simulink model "sampleModel270"  (R2021b)
settings: Solver=VariableStepAuto  StartTime=0.0  StopTime=10.0  RelTol=1e-3
undefined symbols (not defined in the file or in its folder): DiscIntNeverNeededParam, Newton, Raphson
libraries: simulink x19, slpidlib x1
settings Model: Creator=user  LastModifiedBy=user

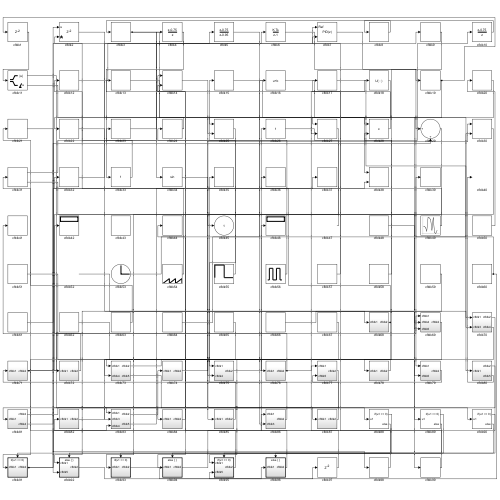
[thumbnail: Simulink's stored preview of the top-level diagram]
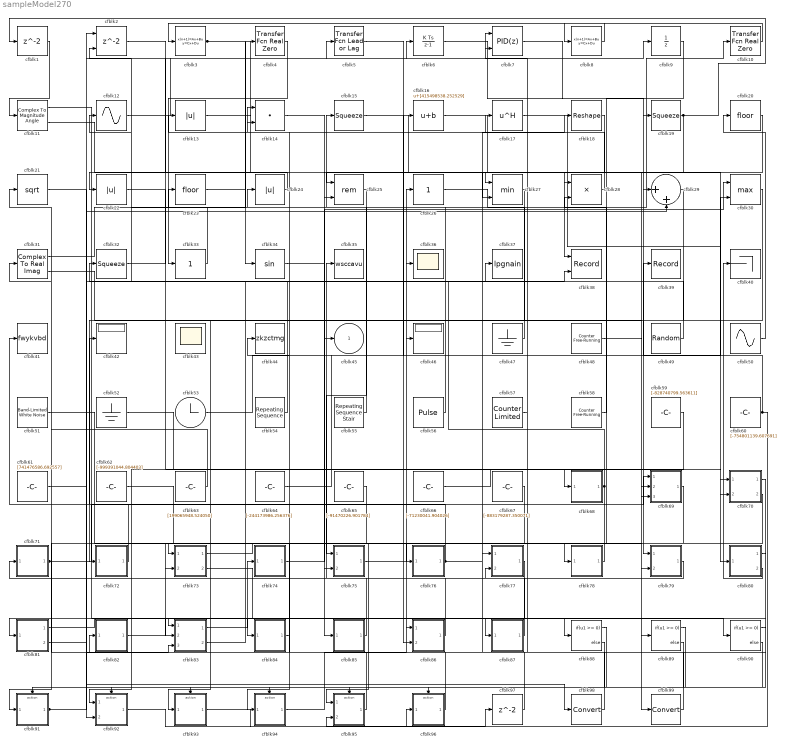
== system sampleModel270 ==
  cfblk1 : Delay  SampleTime=1
  cfblk10 : simulink/Discrete/Transfer Fcn Real Zero  ZeroZ=0.75  ICPrevInput=0.0  DoSatur=off
      settings: SourceProductBaseCode=SL
  cfblk11 : ComplexToMagnitudeAngle
  cfblk12 : Sin  TimeSource=Use external signal  SampleTime=0
  cfblk13 : Abs
  cfblk14 : DotProduct  InputSameDT=on  OutDataTypeStr=Inherit: Inherit via internal rule
  cfblk15 : Squeeze
  cfblk16 : Bias  Bias=[415498538.252529]
  cfblk17 : Math  Operator=hermitian  SaturateOnIntegerOverflow=on
  cfblk18 : Reshape
  cfblk19 : Squeeze
  cfblk2 : Delay  ShowEnablePort=on  SampleTime=1
      settings: InputPortMap=u0,e6
  cfblk20 : Rounding
  cfblk21 : Sqrt  SaturateOnIntegerOverflow=on
  cfblk22 : Abs
  cfblk23 : Rounding
  cfblk24 : Abs
  cfblk25 : Math  Operator=rem  SaturateOnIntegerOverflow=on
  cfblk26 : simulink/Math Operations/Slider Gain  gain=1  low=0  high=2
  cfblk27 : MinMax  Inputs=2
  cfblk28 : Product
  cfblk29 : Sum  Inputs=|++
  cfblk3 : DiscreteStateSpace
  cfblk30 : MinMax  Function=max  Inputs=2
  cfblk31 : ComplexToRealImag
  cfblk32 : Squeeze
  cfblk33 : simulink/Math Operations/Slider Gain  gain=1  low=0  high=2
  cfblk34 : Trigonometry
  cfblk35 : ToWorkspace  VariableName=wsccavu  SaveFormat=Timeseries  SampleTime=-1
  cfblk36 : Scope
  cfblk37 : ToWorkspace  VariableName=lpgnain  SaveFormat=Timeseries  SampleTime=-1
  cfblk38 : Record  FileSettingsInternal="{\"entries\":[{\"content\":{\"excelSettings\":{\"content\":{},\"type\":\"Streamout.ExcelSettings\"}},\"type\":\"Streamout.FileSettingStorage\",\"uuid\":\"55c07847-b416-4147-ba9b-c4fbf5457b55\"}],\"packageUris\":[\"http://schema.mathworks.com/mf0/streamout_blocks/R2020a\"],\"version\":\"1.0\"}"  Layout=[1 1]  SignalsInternal="{\"entries\":[{\"content\":{\"signals\":[{\"content\":{\"blockPath\":[\"sampleModel270/cfblk38\"],\"channel\":[],\"dimensions\":[1],\"domain\":\"sampleModel270/cfblk38\",\"lineColor\":\"#a2142f\",\"plots\":[1],\"port\":1,\"sid\":[\"\"],\"signalID\":11209,\"signalName\":\"cfblk16\"},\"type\":\"RecordBlkView.Signal\",\"uuid\":\"6d9d134b-09a8-4e77-b9a8-4c5e57516884\"},{\"content\":{\"blockPath\":[\"sampleModel270/cfblk38\"],\"channel\":[],\"dimensions\":[1],\"domain\":\"sampleModel270/cfblk38\",\"lineColor\":\"#139fff\",\"plots\":[1],\"port\":2,\"sid\":[\"\"],\"signalID\":11213,\"signalName\":\"cfblk91\"},\"type\":\"RecordBlkView.Signal\",\"uuid\":\"035bce28-8201-4e43-961c-4afa830852dc\"}]},\"type\":\"RecordBlkView.InputSignals\",\"uuid\":\"f20a0d1a-bcdb-4eb4-a0c7-2d20c3785a29\"}],\"packageUris\":[\"http://schema.mathworks.com/mf0/streamout_blocks/R2020a\"],\"version\":\"1.0\"}"  VisualizationBindings="{\"xyplotplugin\":{\"info\":[{\"series\":[{\"bindingParametersList\":[{\"parameter\":\"X-Axis\",\"signalID\":11209,\"signalName\":\"cfblk16\"},{\"parameter\":\"Y-Axis\",\"signalID\":11213,\"signalName\":\"cfblk91\"}],\"seriesID\":19260}],\"subplotID\":1}]}}"  CompatibilityTag=XY
  cfblk39 : Record  FileSettingsInternal="{\"entries\":[{\"content\":{\"excelSettings\":{\"content\":{},\"type\":\"Streamout.ExcelSettings\"}},\"type\":\"Streamout.FileSettingStorage\",\"uuid\":\"3d67d137-5401-4fa9-bcac-a18ba41f64ea\"}],\"packageUris\":[\"http://schema.mathworks.com/mf0/streamout_blocks/R2020a\"],\"version\":\"1.0\"}"  SignalsInternal="{\"entries\":[{\"content\":{\"signals\":[{\"content\":{\"blockPath\":[\"sampleModel270/cfblk39\"],\"channel\":[],\"dimensions\":[1],\"domain\":\"sampleModel270/cfblk39\",\"lineColor\":\"#fe330a\",\"plots\":[1],\"port\":1,\"sid\":[\"\"],\"signalID\":11217,\"signalName\":\"cfblk60\"},\"type\":\"RecordBlkView.Signal\",\"uuid\":\"4590cb18-5316-4242-95f9-f30dc2470911\"}]},\"type\":\"RecordBlkView.InputSignals\",\"uuid\":\"af798ec9-883d-434f-9e97-72437914e7d3\"}],\"packageUris\":[\"http://schema.mathworks.com/mf0/streamout_blocks/R2020a\"],\"version\":\"1.0\"}"  VisualizationBindings="{\"sparklinesplugin\":{\"info\":[{\"bindingParametersList\":[],\"subplotID\":1}]}}"
  cfblk4 : simulink/Discrete/Transfer Fcn Real Zero  ZeroZ=0.75  ICPrevInput=0.0  DoSatur=off
      settings: SourceProductBaseCode=SL
  cfblk40 : Terminator
  cfblk41 : ToWorkspace  VariableName=fwykvbd  SaveFormat=Timeseries  SampleTime=-1
  cfblk42 : Display
  cfblk43 : Scope
      settings: Floating=on
  cfblk44 : ToWorkspace  VariableName=zkzctmg  SaveFormat=Timeseries  SampleTime=-1
  cfblk46 : Display
  cfblk47 : Ground
  cfblk48 : simulink/Sources/Counter Free-Running  NumBits=[30.000000]  tsamp=-1
  cfblk49 : RandomNumber  Mean=[-13361.001595]  Variance=[83852.352686]  Seed=[353484768.000000]  SampleTime=0.1
  cfblk5 : simulink/Discrete/Transfer Fcn Lead or Lag  PoleZ=0.95  ZeroZ=0.75  ICPrevOutput=0.0  ICPrevInput=0.0  DoSatur=off
      settings: SourceProductBaseCode=SL
  cfblk50 : Sin  Amplitude=[595358799.977348]  Bias=[424544015.992801]  SampleTime=0
  cfblk51 : simulink/Sources/Band-Limited White Noise  Cov=[9502367799.789673]  Ts=0.1  seed=[5436201859.000000]
  cfblk52 : Ground
  cfblk53 : Clock
  cfblk54 : simulink/Sources/Repeating Sequence  rep_seq_t=[0 2]  rep_seq_y=[-647210942.038326, -486981734.967450]
  cfblk55 : simulink/Sources/Repeating Sequence Stair  OutValues=[958210710.074239, 342558910.444155]  tsamp=-1  OutMin=[]  OutMax=[]  OutDataTypeStr=double  OutputDataTypeScalingMode=double  OutDataType=fixdt(0,8)  ConRadixGroup=Best Precision: Vector-wise  OutScaling=2^-12
  cfblk56 : DiscretePulseGenerator  PulseType=Time based  Amplitude=[87379413.478695]  Period=[35675365.567741]  PulseWidth=5  PhaseDelay=[7.000000]
  cfblk57 : simulink/Sources/Counter Limited  uplimit=[460.000000]  tsamp=-1
  cfblk58 : simulink/Sources/Counter Free-Running  NumBits=[9.000000]  tsamp=-1
  cfblk59 : Constant  Value=[-828740799.563611]  SampleTime=1
  cfblk6 : DiscreteIntegrator  ICPrevOutput=DiscIntNeverNeededParam  ICPrevScaledInput=DiscIntNeverNeededParam
  cfblk60 : Constant  Value=[-754801139.607691]  SampleTime=1
  cfblk61 : Constant  Value=[741476586.692557]  SampleTime=1
  cfblk62 : Constant  Value=[-999391044.804403]  SampleTime=1
  cfblk63 : Constant  Value=[199065948.524050]  SampleTime=1
  cfblk64 : Constant  Value=[-244173986.256376]  SampleTime=1
  cfblk65 : Constant  Value=[-91470226.901784]  SampleTime=1
  cfblk66 : Constant  Value=[-71230041.904026]  SampleTime=1
  cfblk67 : Constant  Value=[-883179287.350071]  SampleTime=1
  cfblk68 : Subsystem
  cfblk69 : Subsystem
  cfblk7 : slpidlib/PID Controller (2DOF)  Controller=PID  Form=Parallel  TimeDomain=Discrete-time  UseExternalTs=off  SampleTime=1  IntegratorMethod=Forward Euler  FilterMethod=Forward Euler  ControllerParametersSource=internal  P=1  I=1  D=0  UseFilter=on  N=100  b=1  c=1  TunerSelectOption=Transfer Function Based (PID Tuner App)  InitialConditionSource=internal  InitialConditionForIntegrator=0  InitialConditionForFilter=0  DifferentiatorICPrevScaledInput=0  ExternalReset=none  TrackingMode=off  Kt=1  LimitOutput=off  SatLimitsSource=internal  UpperSaturationLimit=inf  LowerSaturationLimit=-inf  LinearizeAsGain=off  AntiWindupMode=none  Kb=1  POutMin=[]  POutMax=[]  IOutMin=[]  IOutMax=[]  DOutMin=[]  DOutMax=[]  NOutMin=[]  NOutMax=[]  bOutMin=[]  bOutMax=[]  cOutMin=[]  cOutMax=[]  SumOutMin=[]  SumOutMax=[]  SaturationOutMin=[]  SaturationOutMax=[]  PParamMin=[]  PParamMax=[]  IParamMin=[]  IParamMax=[]  DParamMin=[]  DParamMax=[]  NParamMin=[]  NParamMax=[]  bParamMin=[]  bParamMax=[]  cParamMin=[]  cParamMax=[]  KbParamMin=[]  KbParamMax=[]  KtParamMin=[]  KtParamMax=[]  KbOutMin=[]  KbOutMax=[]  KtOutMin=[]  KtOutMax=[]  IntegratorOutMin=[]  IntegratorOutMax=[]  FilterOutMin=[]  FilterOutMax=[]  SumI1OutMin=[]  SumI1OutMax=[]  SumI2OutMin=[]  SumI2OutMax=[]  SumI3OutMin=[]  SumI3OutMax=[]  SumI4OutMin=[]  SumI4OutMax=[]  SumDOutMin=[]  SumDOutMax=[]  Sum1OutMin=[]  Sum1OutMax=[]  Sum2OutMin=[]  Sum2OutMax=[]  Sum3OutMin=[]  Sum3OutMax=[]  DifferentiatorOutMin=[]  DifferentiatorOutMax=[]  FilterDiffOutCoefMin=[]  FilterDiffOutCoefMax=[]  ReciprocalOutMin=[]  ReciprocalOutMax=[]  SumDenOutMin=[]  SumDenOutMax=[]  SumNumOutMin=[]  SumNumOutMax=[]  DivideOutMin=[]  DivideOutMax=[]  UdiffTsProdOutMin=[]  UdiffTsProdOutMax=[]  NTsProdOutMin=[]  NTsProdOutMax=[]  UintegralTsProdOutMin=[]  UintegralTsProdOutMax=[]  UngainTsProdOutMin=[]  UngainTsProdOutMax=[]  IntegratorContinuousStateAttributes=''  IntegratorStateMustResolveToSignalObject=off  IntegratorRTWStateStorageClass=Auto  FilterContinuousStateAttributes=''  FilterStateMustResolveToSignalObject=off  FilterRTWStateStorageClass=Auto  ParallelPVariant=InternalParameters  IdealPVariant=Disabled  IVariant=InternalParameters  DVariant=InternalParameters  bVariant=InternalParameters  cVariant=InternalParameters  IntegratorVariant=Discrete  SatVariant=Disabled  AWVariant=Passthrough  PCopyVariant=Disabled  TRVariant=Disabled  FdbkBlocksVariant=Forward  IdealPFdbkVariant=Disabled  SatFdbkVariant=Disabled  DerivativeFilterVariant=ForwardEulerFilter  NVariant=InternalParameters  NCopyVariant=Disabled  FilterICVariant=InternalICsFilter  IntegratorICVariant=InternalICs  ExternalResetVariant=Disabled  TRSumVariant=Passthrough  SumFdbkVariant=Disabled  SumVariant=Sum_PID  TsampFilterVariant=InternalTs  TsampNgainVariant=Passthrough  TsampIntegralVariant=Passthrough  ExternalSaturationOutDataTypeStr=Inherit: Same as second input
      settings: SourceProductBaseCode=SL
  cfblk70 : Subsystem
  cfblk71 : Subsystem
  cfblk72 : Subsystem
  cfblk73 : Subsystem
  cfblk74 : Subsystem
  cfblk75 : Subsystem
  cfblk76 : Subsystem
  cfblk77 : Subsystem
  cfblk78 : Subsystem
  cfblk79 : Subsystem
  cfblk8 : DiscreteStateSpace
  cfblk80 : Subsystem
  cfblk81 : Subsystem
  cfblk82 : Subsystem
  cfblk83 : Subsystem
  cfblk84 : Subsystem
  cfblk85 : Subsystem
  cfblk86 : Subsystem
  cfblk87 : Subsystem
  cfblk88 : If  IfExpression=u1 >= 0  SampleTime=1
  cfblk89 : If  IfExpression=u1 >= 0  SampleTime=1
  cfblk9 : UnitDelay  HasFrameUpgradeWarning=on
  cfblk90 : If  IfExpression=u1 >= 0  SampleTime=1
  cfblk91 : Subsystem  TreatAsAtomicUnit=on
  cfblk92 : Subsystem  TreatAsAtomicUnit=on
  cfblk93 : Subsystem  TreatAsAtomicUnit=on
  cfblk94 : Subsystem  TreatAsAtomicUnit=on
  cfblk95 : Subsystem  TreatAsAtomicUnit=on
  cfblk96 : Subsystem  TreatAsAtomicUnit=on
  cfblk97 : Delay  SampleTime=1
  cfblk98 : DataTypeConversion
  cfblk99 : DataTypeConversion
  cfblk45 : Outport
  wires:
  cfblk3/1 -> cfblk27/1, cfblk25/2
  cfblk11/1 -> cfblk84/1(cfblk1)
  cfblk49/1 -> cfblk32/1
  cfblk8/1 -> cfblk3/1
  cfblk70/1(cfblk2) -> cfblk82/1(cfblk1)
  cfblk86/1(cfblk2) -> cfblk35/1
  cfblk83/1(cfblk2) -> cfblk74/1(cfblk1)
  cfblk80/1(cfblk2) -> cfblk81/1(cfblk1)
  cfblk72/1(cfblk2) -> cfblk41/1
  cfblk56/1 -> cfblk15/1
  cfblk26/1 -> cfblk10/1
  cfblk55/1 -> cfblk24/1
  cfblk16/1 -> cfblk38/1
  cfblk85/1(cfblk2) -> cfblk71/1(cfblk1)
  cfblk80/2(cfblk5) -> cfblk40/1
  cfblk54/1 -> cfblk12/1
  cfblk9/1 -> cfblk78/1(cfblk1)
  cfblk12/1 -> cfblk6/1
  cfblk59/1 -> cfblk92/1(cfblk1)
  cfblk96/1(cfblk2) -> cfblk26/1
  cfblk4/1 -> cfblk33/1
  cfblk28/1 -> cfblk13/1
  cfblk87/1(cfblk2) -> cfblk14/1
  cfblk84/1(cfblk2) -> cfblk44/1
  cfblk25/1 -> cfblk75/1(cfblk1)
  cfblk77/1(cfblk2) -> cfblk92/2(cfblk5)
  cfblk15/1 -> cfblk70/1(cfblk1)
  cfblk6/1 -> cfblk79/1(cfblk1)
  cfblk69/1(cfblk2) -> cfblk95/1(cfblk1)
  cfblk23/1 -> cfblk9/1
  cfblk74/1(cfblk2) -> cfblk30/1
  cfblk17/1 -> cfblk80/1(cfblk1)
  cfblk83/2(cfblk5) -> cfblk37/1
  cfblk32/1 -> cfblk7/1
  cfblk75/1(cfblk2) -> cfblk46/1
  cfblk79/1(cfblk2) -> cfblk77/2(cfblk5)
  cfblk73/1(cfblk2) -> cfblk76/1(cfblk1)
  cfblk60/1 -> cfblk95/2(cfblk5), cfblk39/1
  cfblk10/1 -> cfblk8/1
  cfblk94/1(cfblk2) -> cfblk86/1(cfblk1)
  cfblk50/1 -> cfblk20/1
  cfblk71/1(cfblk2) -> cfblk69/1(cfblk1), cfblk29/2
  cfblk47/1 -> cfblk23/1
  cfblk34/1 -> cfblk45/1
  cfblk93/1(cfblk2) -> cfblk96/1(cfblk1)
  cfblk18/1 -> cfblk27/2
  cfblk22/1 -> cfblk70/2(cfblk3)
  cfblk1/1 -> cfblk11/1
  cfblk53/1 -> cfblk16/1
  cfblk7/1 -> cfblk19/1
  cfblk68/1(cfblk2) -> cfblk36/1, cfblk73/2(cfblk4)
  cfblk27/1 -> cfblk75/2(cfblk4)
  cfblk5/1 -> cfblk90/1
  cfblk78/1(cfblk2) -> cfblk73/1(cfblk1)
  cfblk14/1 -> cfblk86/2(cfblk3)
  cfblk70/2(cfblk4) -> cfblk91/1(cfblk1)
  cfblk19/1 -> cfblk1/1, cfblk25/1
  cfblk73/2(cfblk5) -> cfblk87/1(cfblk1)
  cfblk63/1 -> cfblk31/1
  cfblk67/1 -> cfblk94/1(cfblk1)
  cfblk2/1 -> cfblk28/1
  cfblk66/1 -> cfblk69/2(cfblk4)
  cfblk20/1 -> cfblk69/3(cfblk5)
  cfblk81/1(cfblk2) -> cfblk83/1(cfblk1)
  cfblk65/1 -> cfblk83/2(cfblk3)
  cfblk91/1(cfblk2) -> cfblk83/3(cfblk4), cfblk38/2
  cfblk31/1 -> cfblk4/1
  cfblk51/1 -> cfblk79/2(cfblk5)
  cfblk24/1 -> cfblk22/1
  cfblk52/1 -> cfblk68/1(cfblk1)
  cfblk13/1 -> cfblk29/1
  cfblk76/1(cfblk2) -> cfblk18/1, cfblk42/1
  cfblk61/1 -> cfblk2/1
  cfblk31/2 -> cfblk89/1
  cfblk95/1(cfblk2) -> cfblk14/2
  cfblk64/1 -> cfblk30/2
  cfblk29/1 -> cfblk93/1(cfblk1)
  cfblk82/1(cfblk2) -> cfblk88/1
  cfblk57/1 -> cfblk7/2
  cfblk81/2(cfblk4) -> cfblk5/1
  cfblk58/1 -> cfblk28/2
  cfblk62/1 -> cfblk85/1(cfblk1)
  cfblk30/1 -> cfblk72/1(cfblk1)
  cfblk33/1 -> cfblk2/2
  cfblk11/2 -> cfblk34/1
  cfblk88/1 -> cfblk91/Action
  cfblk88/2 -> cfblk92/Action
  cfblk89/1 -> cfblk93/Action
  cfblk89/2 -> cfblk94/Action
  cfblk90/1 -> cfblk95/Action
  cfblk90/2 -> cfblk96/Action
  cfblk92/1(cfblk2) -> cfblk97/1
  cfblk97/1 -> cfblk77/1(cfblk1)
  cfblk21/1 -> cfblk98/1
  cfblk98/1 -> cfblk17/1
  cfblk48/1 -> cfblk99/1
  cfblk99/1 -> cfblk21/1

== system sampleModel270/cfblk68 ==
  cfblk1 : Inport
  cfblk3 : DiscreteFir  SampleTime=1
  cfblk2 : Outport
  wires:
  cfblk1/1 -> cfblk3/1
  cfblk3/1 -> cfblk2/1

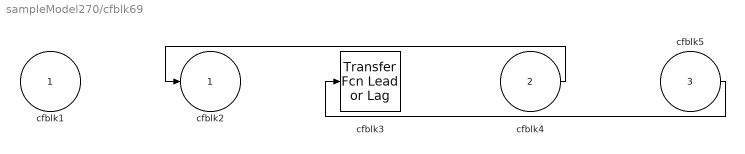
== system sampleModel270/cfblk69 ==
  cfblk1 : Inport
  cfblk4 : Inport  Port=2
  cfblk5 : Inport  Port=3
  cfblk3 : simulink/Discrete/Transfer Fcn Lead or Lag  PoleZ=0.95  ZeroZ=0.75  ICPrevOutput=0.0  ICPrevInput=0.0  DoSatur=off
      settings: SourceProductBaseCode=SL
  cfblk2 : Outport
  wires:
  cfblk4/1 -> cfblk2/1
  cfblk5/1 -> cfblk3/1

== system sampleModel270/cfblk70 ==
  cfblk1 : Inport
  cfblk3 : Inport  Port=2
  cfblk2 : Outport
  cfblk4 : Outport  Port=2
  wires:
  cfblk1/1 -> cfblk2/1
  cfblk3/1 -> cfblk4/1

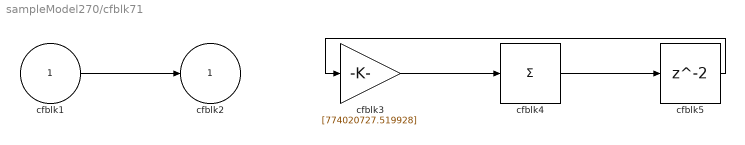
== system sampleModel270/cfblk71 ==
  cfblk1 : Inport
  cfblk3 : Gain  Gain=[774020727.519928]
  cfblk4 : Sum  Inputs=+
  cfblk5 : Delay  SampleTime=1
  cfblk2 : Outport
  wires:
  cfblk3/1 -> cfblk4/1
  cfblk1/1 -> cfblk2/1
  cfblk4/1 -> cfblk5/1
  cfblk5/1 -> cfblk3/1

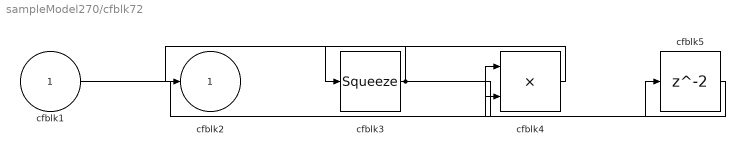
== system sampleModel270/cfblk72 ==
  cfblk1 : Inport
  cfblk3 : Squeeze
  cfblk4 : Product
  cfblk5 : Delay  SampleTime=1
  cfblk2 : Outport
  wires:
  cfblk4/1 -> cfblk3/1
  cfblk1/1 -> cfblk4/1
  cfblk3/1 -> cfblk2/1, cfblk5/1
  cfblk5/1 -> cfblk4/2

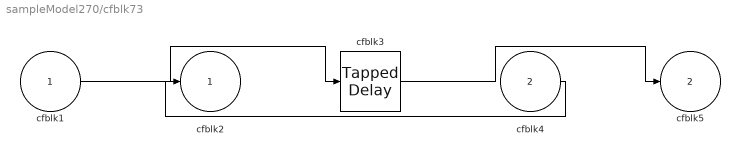
== system sampleModel270/cfblk73 ==
  cfblk1 : Inport
  cfblk4 : Inport  Port=2
  cfblk3 : simulink/Discrete/Tapped Delay  vinit=0.0  samptime=-1  NumDelays=1  DelayOrder=Oldest  includeCurrent=off
  cfblk2 : Outport
  cfblk5 : Outport  Port=2
  wires:
  cfblk1/1 -> cfblk3/1
  cfblk4/1 -> cfblk2/1
  cfblk3/1 -> cfblk5/1

== system sampleModel270/cfblk74 ==
  cfblk1 : Inport
  cfblk3 : DiscreteStateSpace
  cfblk2 : Outport
  wires:
  cfblk1/1 -> cfblk3/1
  cfblk3/1 -> cfblk2/1

== system sampleModel270/cfblk75 ==
  cfblk1 : Inport
  cfblk4 : Inport  Port=2
  cfblk3 : Polyval  Coefs=[ +2.081618890e-019, -1.441693666e-014, +4.719686976e-010, -8.536869453e-006, +1.621573104e-001, -8.087801117e+001 ]
  cfblk2 : Outport
  wires:
  cfblk3/1 -> cfblk2/1
  cfblk4/1 -> cfblk3/1

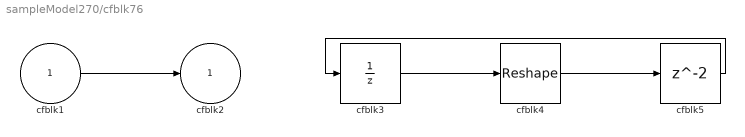
== system sampleModel270/cfblk76 ==
  cfblk1 : Inport
  cfblk3 : UnitDelay  HasFrameUpgradeWarning=on
  cfblk4 : Reshape
  cfblk5 : Delay  SampleTime=1
  cfblk2 : Outport
  wires:
  cfblk3/1 -> cfblk4/1
  cfblk1/1 -> cfblk2/1
  cfblk4/1 -> cfblk5/1
  cfblk5/1 -> cfblk3/1

== system sampleModel270/cfblk77 ==
  cfblk1 : Inport
  cfblk5 : Inport  Port=2
  cfblk3 : Product  Inputs=**
  cfblk4 : Constant  Value=[-653733544.862791]  SampleTime=1
  cfblk2 : Outport
  wires:
  cfblk5/1 -> cfblk3/1
  cfblk4/1 -> cfblk2/1
  cfblk1/1 -> cfblk3/2

== system sampleModel270/cfblk78 ==
  cfblk1 : Inport
  cfblk3 : DiscreteZeroPole  Poles=[0 0.5]  Gain=1
  cfblk4 : Constant  Value=[-229940139.054615]  SampleTime=1
  cfblk2 : Outport
  wires:
  cfblk1/1 -> cfblk2/1
  cfblk4/1 -> cfblk3/1

== system sampleModel270/cfblk79 ==
  cfblk1 : Inport
  cfblk5 : Inport  Port=2
  cfblk3 : DiscreteStateSpace
  cfblk4 : ComplexToRealImag
  cfblk2 : Outport
  wires:
  cfblk5/1 -> cfblk4/1
  cfblk1/1 -> cfblk3/1
  cfblk4/1 -> cfblk2/1

== system sampleModel270/cfblk80 ==
  cfblk1 : Inport
  cfblk3 : Delay  SampleTime=1
  cfblk4 : Sum  Inputs=|++
  cfblk2 : Outport
  cfblk5 : Outport  Port=2
  wires:
  cfblk3/1 -> cfblk5/1, cfblk4/1, cfblk4/2
  cfblk1/1 -> cfblk3/1
  cfblk4/1 -> cfblk2/1

== system sampleModel270/cfblk81 ==
  cfblk1 : Inport
  cfblk3 : Trigonometry
  cfblk2 : Outport
  cfblk4 : Outport  Port=2
  wires:
  cfblk3/1 -> cfblk2/1
  cfblk1/1 -> cfblk3/1, cfblk4/1

== system sampleModel270/cfblk82 ==
  cfblk1 : Inport
  cfblk3 : Constant  Value=[966089803.831900]  SampleTime=1
  cfblk2 : Outport
  wires:
  cfblk3/1 -> cfblk2/1

== system sampleModel270/cfblk83 ==
  cfblk1 : Inport
  cfblk3 : Inport  Port=2
  cfblk4 : Inport  Port=3
  cfblk2 : Outport
  cfblk5 : Outport  Port=2
  wires:
  cfblk3/1 -> cfblk2/1
  cfblk1/1 -> cfblk5/1

== system sampleModel270/cfblk84 ==
  cfblk1 : Inport
  cfblk3 : DiscreteTransferFcn  SampleTime=1
  cfblk4 : DiscreteIntegrator  ICPrevOutput=DiscIntNeverNeededParam  ICPrevScaledInput=DiscIntNeverNeededParam
  cfblk2 : Outport
  wires:
  cfblk1/1 -> cfblk3/1
  cfblk4/1 -> cfblk2/1
  cfblk3/1 -> cfblk4/1

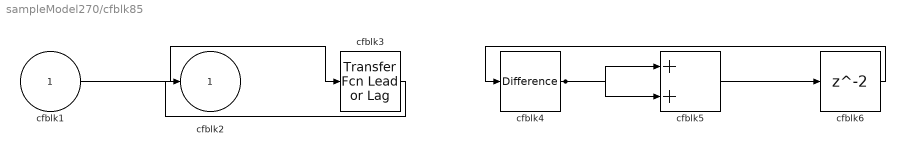
== system sampleModel270/cfblk85 ==
  cfblk1 : Inport
  cfblk3 : simulink/Discrete/Transfer Fcn Lead or Lag  PoleZ=0.95  ZeroZ=0.75  ICPrevOutput=0.0  ICPrevInput=0.0  DoSatur=off
      settings: SourceProductBaseCode=SL
  cfblk4 : simulink/Discrete/Difference  ICPrevInput=0.0  OutMin=[]  OutMax=[]  OutDataTypeStr=Inherit: Inherit via back propagation  OutDataType=fixdt(1, 16)  OutScaling=2^-10  DoSatur=off
  cfblk5 : Sum
  cfblk6 : Delay  SampleTime=1
  cfblk2 : Outport
  wires:
  cfblk1/1 -> cfblk3/1
  cfblk4/1 -> cfblk5/1, cfblk5/2
  cfblk3/1 -> cfblk2/1
  cfblk5/1 -> cfblk6/1
  cfblk6/1 -> cfblk4/1

== system sampleModel270/cfblk86 ==
  cfblk1 : Inport
  cfblk3 : Inport  Port=2
  cfblk2 : Outport
  wires:
  cfblk1/1 -> cfblk2/1

== system sampleModel270/cfblk87 ==
  cfblk1 : Inport
  cfblk3 : DotProduct  InputSameDT=on  OutDataTypeStr=Inherit: Inherit via internal rule
  cfblk4 : simulink/Math Operations/MinMax Running Resettable  Function=min  vinit=0.0
  cfblk5 : Delay  SampleTime=1
  cfblk2 : Outport
  wires:
  cfblk1/1 -> cfblk4/1, cfblk3/2
  cfblk4/1 -> cfblk3/1
  cfblk3/1 -> cfblk2/1, cfblk5/1
  cfblk5/1 -> cfblk4/2

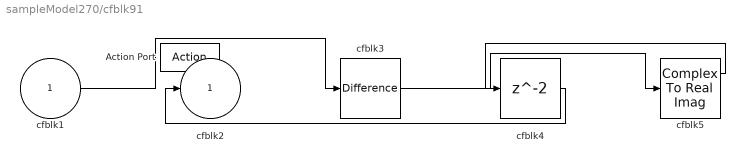
== system sampleModel270/cfblk91 ==
  cfblk1 : Inport
  Action Port : ActionPort  ActionPortLabel=if(u1 >= 0)
  cfblk3 : simulink/Discrete/Difference  ICPrevInput=0.0  OutMin=[]  OutMax=[]  OutDataTypeStr=Inherit: Inherit via back propagation  OutDataType=fixdt(1, 16)  OutScaling=2^-10  DoSatur=off
  cfblk4 : Delay
  cfblk5 : ComplexToRealImag
  cfblk2 : Outport
  wires:
  cfblk4/1 -> cfblk2/1
  cfblk1/1 -> cfblk3/1
  cfblk3/1 -> cfblk5/1
  cfblk5/1 -> cfblk4/1

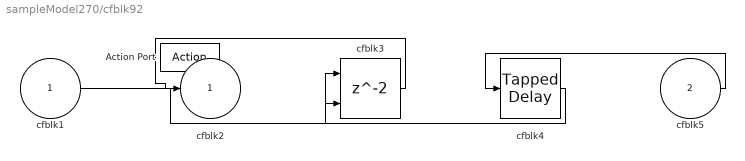
== system sampleModel270/cfblk92 ==
  cfblk1 : Inport
  cfblk5 : Inport  Port=2
  Action Port : ActionPort  ActionPortLabel=else
  cfblk3 : Delay  ShowEnablePort=on
      settings: InputPortMap=u0,e6
  cfblk4 : simulink/Discrete/Tapped Delay  vinit=0.0  samptime=-1  NumDelays=1  DelayOrder=Oldest  includeCurrent=off
  cfblk2 : Outport
  wires:
  cfblk1/1 -> cfblk3/1
  cfblk5/1 -> cfblk4/1
  cfblk4/1 -> cfblk3/2
  cfblk3/1 -> cfblk2/1

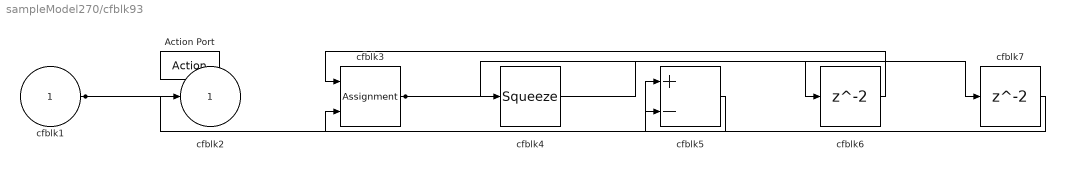
== system sampleModel270/cfblk93 ==
  cfblk1 : Inport
  Action Port : ActionPort  ActionPortLabel=if(u1 >= 0)
  cfblk3 : Assignment  DiagnosticForDimensions=Warning  IndexOptions=Index vector (dialog)  Indices=1  OutputSizes=1
  cfblk4 : Squeeze
  cfblk5 : Sum  Inputs=+-
  cfblk6 : Delay
  cfblk7 : Delay
  cfblk2 : Outport
  wires:
  cfblk1/1 -> cfblk2/1, cfblk5/1
  cfblk3/1 -> cfblk4/1, cfblk7/1
  cfblk5/1 -> cfblk3/2
  cfblk4/1 -> cfblk6/1
  cfblk6/1 -> cfblk3/1
  cfblk7/1 -> cfblk5/2

== system sampleModel270/cfblk94 ==
  cfblk1 : Inport
  Action Port : ActionPort  ActionPortLabel=else
  cfblk3 : DiscreteStateSpace  SampleTime=-1
  cfblk4 : Sqrt  Operator=rSqrt  AlgorithmType=Newton-Raphson  SaturateOnIntegerOverflow=on
  cfblk2 : Outport
  wires:
  cfblk1/1 -> cfblk4/1
  cfblk4/1 -> cfblk3/1
  cfblk3/1 -> cfblk2/1

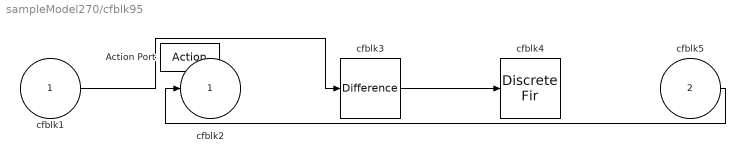
== system sampleModel270/cfblk95 ==
  cfblk1 : Inport
  cfblk5 : Inport  Port=2
  Action Port : ActionPort  ActionPortLabel=if(u1 >= 0)
  cfblk3 : simulink/Discrete/Difference  ICPrevInput=0.0  OutMin=[]  OutMax=[]  OutDataTypeStr=Inherit: Inherit via back propagation  OutDataType=fixdt(1, 16)  OutScaling=2^-10  DoSatur=off
  cfblk4 : DiscreteFir
  cfblk2 : Outport
  wires:
  cfblk5/1 -> cfblk2/1
  cfblk1/1 -> cfblk3/1
  cfblk3/1 -> cfblk4/1

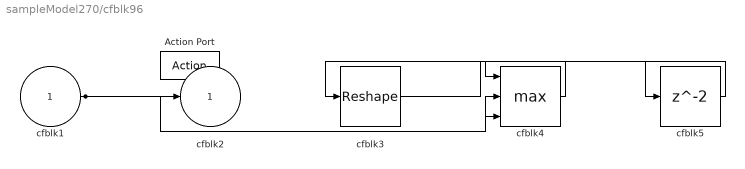
== system sampleModel270/cfblk96 ==
  cfblk1 : Inport
  Action Port : ActionPort  ActionPortLabel=else
  cfblk3 : Reshape
  cfblk4 : MinMax  Function=max  Inputs=3
  cfblk5 : Delay
  cfblk2 : Outport
  wires:
  cfblk1/1 -> cfblk2/1, cfblk4/2, cfblk4/3
  cfblk4/1 -> cfblk3/1
  cfblk3/1 -> cfblk5/1
  cfblk5/1 -> cfblk4/1
